simulink model "Model_Simulation"  (R2016a)
settings: Solver=FixedStepAuto  StartTime=0.0  StopTime=5  FixedStep=2e-6  RelTol=1e-3
values from neighbouring files (symbols this model uses):
  C = 3060e-6    (= 0.00306)    [Controle_Inversor_UR_D.m]
  Ki_i_disc = wc*Rf    (= 44.2477838534)    [Controle_Inversor_UR_D.m]
  Ki_i_disc_b = wc_b*Rb/Vdc    (= 0.0983284085631)    [Controle_Inversor_UR_D.m]
  Ki_q_disc = wq/H    [Controle_Inversor_UR_D.m]
  Ki_v_disc_b = wc_bv/Req    (= 14.5799013102)    [Controle_Inversor_UR_D.m]
  Ki_vdc_disc = ((wvdc)^2*C)/Gt    [Controle_Inversor_UR_D.m]
  Kp_i_disc = wc*Lf    (= 2.19688771906)    [Controle_Inversor_UR_D.m]
  Kp_i_disc_b = wc_b*Lb/Vdc    (= 0.00545604673435)    [Controle_Inversor_UR_D.m]
  Kp_q_disc = Ki_q_disc*(Lf/Kp_i_disc)    [Controle_Inversor_UR_D.m]
  Kp_v_disc_b = wc_bv*Cin    (= 0.0356301510224)    [Controle_Inversor_UR_D.m]
  Kp_vdc_disc = (2*ksi_vdc*wvdc*C)/Gt    [Controle_Inversor_UR_D.m]
  Lf = (0.0012+2.8949e-04)    (= 0.00148949)    [Controle_Inversor_UR_D.m]
  Tsw = 1/fsw    (= 0.0002)    [Controle_Inversor_UR_D.m]
  w = 2*pi*60    (= 376.991118431)    [Controle_Inversor_UR_D.m]
undefined symbols (not defined in the file or in its folder): D1, dEgdT, Delta, EgRef, gcbh, k1, Rsh_array5pc, sigbuilder_block, sps_rtmsupport, Tref_K, VT_ref
libraries: powerlib x179, simulink x14, powerlib_meascontrol x13, spsPVarrayModel x12
(part 15 of 20)

== system Model_Simulation/Subsystem2/Conversor Boost Fotovoltaico2 ==
  PWM : Inport
  Arranjo 8 strings em paralelo com 43 módulos em série Vmp = 43 x 30,6 = 1315,8 V Imp = 8,32 x 7 = 58,24 A 76.632,192 W : Subsystem  AncestorBlock=re_lib/Solar/PV Array  DialogController=POWERSYS.PowerSysDialog  LoadFcn=sps_rtmsupport('LoadFcn',gcbh);  StartFcn=sps_rtmsupport('StartFcn',gcbh);  StopFcn=sps_rtmsupport('StopFcn',gcbh);  mask(PV array){Npar=7, Nser=43, PlotType=array @ 25 deg.C & specified irradiances, S_vec=[ 1000  500  100 ], Temp_C_vec=[ 45 25  ], ModuleName=Yingli Energy (China) YL255P-29b, PlotWhenSelected=off, Pm=254.592, Ncell=60, Voc=38.7, Isc=8.88, Vm=30.6, Im=8.32, beta_Voc_pc=-0.337, alpha_Isc_pc=0.043795, beta_Voc=-0.13042, alpha_Isc=0.003889, IL=8.9, I0=1.2854e-10, nI=1.0063, Rsh=310.1051, Rs=0.42879, BAL=on, Tc=1e-7, Tfilter=5e-5}
      mask prompts: Npar "Parallel strings"; Nser "Series-connected modules per string"; S_vec "Irradiances (W/m2)"; Temp_C_vec "T_cell (deg. C)"; ModuleName "Module:"; PlotWhenSelected "Plot I-V and P-V characteristics when a module is selected"; Pm "Maximum Power (W)"; Ncell "Cells per module (Ncell)"; Voc "Open circuit voltage  Voc (V)"; Isc "Short-circuit current Isc (A)"; Vm "Voltage at maximum power point Vmp (V)"; Im "Current at maximum power point Imp (A)"; beta_Voc_pc "Temperature coefficient of Voc (%/deg.C)"; alpha_Isc_pc "Temperature coefficient of Isc (%/deg.C)"; beta_Voc "Temperature coefficient of Voc (V/deg.C)"; alpha_Isc "Temperature coefficient of Isc (A/deg.C)"; IL "Light-generated current IL (A)"; I0 "Diode saturation current I0 (A)"; nI "Diode ideality factor"; Rsh "Shunt resistance Rsh (ohms)"; Rs "Series resistance Rs (ohms)"; BAL "Break algebaic loop in internal model"; Tc "Time constant (s)"; Tfilter "Time constant (s)"
      mask help:
      | Implements a PV array built of strings of PV modules connected in parallel. Each string consists of modules connected in series.
      | Allows modeling of a variety of preset PV modules available from NREL System Advisor Model (Jan. 2014) as well as user-defined PV module.
      |
      | Input 1 = Sun irradiance, in W/m2, and input 2 = Cell temperature, in deg.C.
      mask init: same as Model_Simulation/Subsystem2/Arranjo 21 strings em paralelo com 43 módulos em série Vmp = 43 x 30,6 = 1315,8 V Imp = 8,32 x 21 = 174,72 A 229.896,576 W
      settings: CopyFcn=sps_rtmsupport('CopyFcn',gcbh);  DeleteFcn=sps_rtmsupport('DeleteFcn',gcbh);  UndoDeleteFcn=sps_rtmsupport('UndoDeleteFcn',gcbh);  ModelCloseFcn=sps_rtmsupport('ModelCloseFcn',gcbh);  PreSaveFcn=sps_rtmsupport('PreSaveFcn',gcbh);  PostSaveFcn=sps_rtmsupport('PostSaveFcn',gcbh);  NameChangeFcn=sps_rtmsupport('NameChangeFcn',gcbh);  PreCopyFcn=sps_rtmsupport('PreCopyFcn',gcbh);  CloseFcn=sps_rtmsupport('CloseFcn',gcbh);  PreDeleteFcn=sps_rtmsupport('PreDeleteFcn',gcbh);
      settings: OpenFcn=|
      | %assignin('base','PVMaskOpening',1);
      | %open_system(gcb,'mask')
      | %assignin('base','PVMaskOpening',0);
      | sps_rtmsupport('OpenFcn',gcbh, [3 6 7 23]);
      mask Help: helpview(psbhelp);
      mask TypeOptions PlotType: one module @ 25 deg.C & specified irradiances | array @ 25 deg.C & specified irradiances | array @ 1000 W/m2 & specified temperatures
      mask Callback PlotType: PVArrayCback(gcb)
